simulink model "zadanie5sim"  (R2025b)
settings: Solver=VariableStepAuto  StartTime=0.0  StopTime=100  RelTol=1e-3
values from neighbouring files (symbols this model uses):
  dsys = c2d(sys, 0.1)    [zadanie5.m]
  I = 15    [zadanie4.m]    (also in zadanie5.m = 0)
  P = 100    [zadanie4.m]    (also in zadanie5.m = 17)
settings Model: Creator=micha  LastModifiedBy=Michał

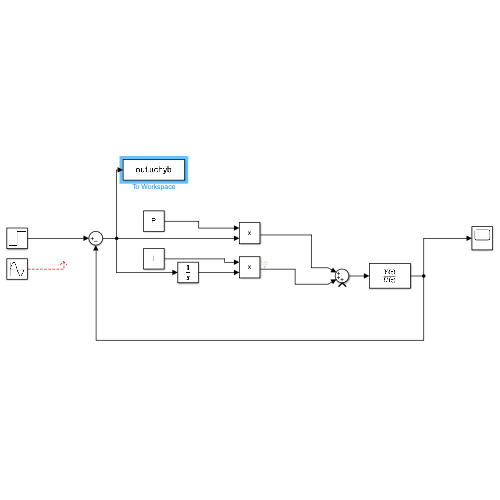
[thumbnail: Simulink's stored preview of the top-level diagram]
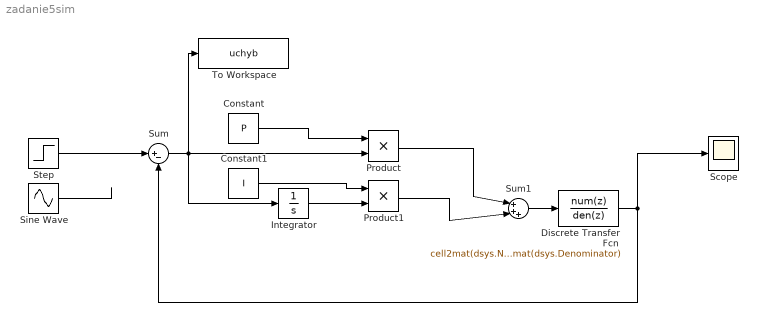
== system zadanie5sim ==
  Constant : Constant  Value=P
  Constant1 : Constant  Value=I  SampleTime=0
  Discrete Transfer Fcn : DiscreteTransferFcn  Numerator=cell2mat(dsys.Numerator)  Denominator=cell2mat(dsys.Denominator)
  Integrator : Integrator
  Product : Product
  Product1 : Product
  Scope : Scope
      settings: SampleTime=0.01  ActiveDisplayYMinimum=-0.1062372201911924  ActiveDisplayYMaximum=0.95613498172073186
  Sine Wave : Sin  Frequency=0.005  SampleTime=0
  Step : Step  SampleTime=0
  Sum : Sum  Inputs=|+-
  Sum1 : Sum  Inputs=|+++
  To Workspace : ToWorkspace  VariableName=uchyb  SampleTime=-1
      settings: Save2DSignal=2-D array (concatenate along first dimension)
  wires:
  Step/1 -> Sum/1
  Sum/1 -> To Workspace/1, Integrator/1, Product/2
  Sum1/1 -> Discrete Transfer Fcn/1
  Constant/1 -> Product/1
  Product/1 -> Sum1/1
  Integrator/1 -> Product1/2
  Product1/1 -> Sum1/2
  Constant1/1 -> Product1/1
  Sine Wave/1 -> ?
  Discrete Transfer Fcn/1 -> Scope/1, Sum/2
